simulink library "rangeSensorState"  (R2017b)
settings: Solver=VariableStepAuto  StartTime=0.0  StopTime=10.0  RelTol=1e-3
settings Model: Creator=Hoa  LastModifiedBy=Hoa

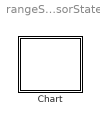
== system rangeSensorState ==
  Chart : Stateflow chart  TreatAsAtomicUnit=on

== stateflow chart rangeSensorState/Chart ==
  state ?
  (default) -> ?
